simulink model "c00021M_harness"  (R2018a)
settings: Solver=ode3  StartTime=0.0  StopTime=10.0  RelTol=1e-3  EnableMultiTasking=on
undefined symbols (not defined in the file): b, DiscIntNeverNeededParam, J, K, L, PosMinimaW3, R, sigbuilder_block
(part 36 of 45)

== system c00021M_harness/M171/Physical/W/DC_Engine ==
  input : Inport
  (Inductance) : Gain  Gain=1/L
  (Inductance)1 : Gain  Gain=1/J
  Add : Sum  Inputs=-+-
  Add1 : Sum  Inputs=+-
  Damping : Gain  Gain=b
  Discrete-Time Integrator : DiscreteIntegrator  SampleTime=-1  ICPrevOutput=DiscIntNeverNeededParam  ICPrevScaledInput=DiscIntNeverNeededParam
  Discrete-Time Integrator1 : DiscreteIntegrator  SampleTime=-1  ICPrevOutput=DiscIntNeverNeededParam  ICPrevScaledInput=DiscIntNeverNeededParam
  Ke : Gain  Gain=K
  Kt : Gain  Gain=K
  Resistance : Gain  Gain=R
  Voltage : Gain  Gain=10
  Speed : Outport
  wires:
  (Inductance)/1 -> Discrete-Time Integrator/1
  Damping/1 -> Add1/2
  Discrete-Time Integrator1/1 -> Damping/1, Speed/1, Ke/1
  (Inductance)1/1 -> Discrete-Time Integrator1/1
  Add1/1 -> (Inductance)1/1
  Kt/1 -> Add1/1
  Ke/1 -> Add/3
  Resistance/1 -> Add/1
  Discrete-Time Integrator/1 -> Resistance/1, Kt/1
  Add/1 -> (Inductance)/1
  Voltage/1 -> Add/2
  input/1 -> Voltage/1

== system c00021M_harness/M171/Physical/W5/DC_Engine ==
  input : Inport
  (Inductance) : Gain  Gain=1/L
  (Inductance)1 : Gain  Gain=1/J
  Add : Sum  Inputs=-+-
  Add1 : Sum  Inputs=+-
  Damping : Gain  Gain=b
  Discrete-Time Integrator : DiscreteIntegrator  SampleTime=-1  ICPrevOutput=DiscIntNeverNeededParam  ICPrevScaledInput=DiscIntNeverNeededParam
  Discrete-Time Integrator1 : DiscreteIntegrator  SampleTime=-1  ICPrevOutput=DiscIntNeverNeededParam  ICPrevScaledInput=DiscIntNeverNeededParam
  Ke : Gain  Gain=K
  Kt : Gain  Gain=K
  Resistance : Gain  Gain=R
  Voltage : Gain  Gain=10
  Speed : Outport
  wires:
  input/1 -> Voltage/1
  Voltage/1 -> Add/2
  Add/1 -> (Inductance)/1
  (Inductance)/1 -> Discrete-Time Integrator/1
  Discrete-Time Integrator/1 -> Kt/1, Resistance/1
  Resistance/1 -> Add/1
  Ke/1 -> Add/3
  Kt/1 -> Add1/1
  Add1/1 -> (Inductance)1/1
  (Inductance)1/1 -> Discrete-Time Integrator1/1
  Discrete-Time Integrator1/1 -> Ke/1, Speed/1, Damping/1
  Damping/1 -> Add1/2

== system c00021M_harness/M171/Physical/W6/DC_Engine ==
  input : Inport
  (Inductance) : Gain  Gain=1/L
  (Inductance)1 : Gain  Gain=1/J
  Add : Sum  Inputs=-+-
  Add1 : Sum  Inputs=+-
  Damping : Gain  Gain=b
  Discrete-Time Integrator : DiscreteIntegrator  SampleTime=-1  ICPrevOutput=DiscIntNeverNeededParam  ICPrevScaledInput=DiscIntNeverNeededParam
  Discrete-Time Integrator1 : DiscreteIntegrator  SampleTime=-1  ICPrevOutput=DiscIntNeverNeededParam  ICPrevScaledInput=DiscIntNeverNeededParam
  Ke : Gain  Gain=K
  Kt : Gain  Gain=K
  Resistance : Gain  Gain=R
  Voltage : Gain  Gain=10
  Speed : Outport
  wires:
  Damping/1 -> Add1/2
  Discrete-Time Integrator1/1 -> Damping/1, Speed/1, Ke/1
  (Inductance)1/1 -> Discrete-Time Integrator1/1
  Add1/1 -> (Inductance)1/1
  Kt/1 -> Add1/1
  Ke/1 -> Add/3
  Resistance/1 -> Add/1
  Discrete-Time Integrator/1 -> Resistance/1, Kt/1
  (Inductance)/1 -> Discrete-Time Integrator/1
  Add/1 -> (Inductance)/1
  Voltage/1 -> Add/2
  input/1 -> Voltage/1

== system c00021M_harness/M172/Physical/W/DC_Engine ==
  input : Inport
  (Inductance) : Gain  Gain=1/L
  (Inductance)1 : Gain  Gain=1/J
  Add : Sum  Inputs=-+-
  Add1 : Sum  Inputs=+-
  Damping : Gain  Gain=b
  Discrete-Time Integrator : DiscreteIntegrator  SampleTime=-1  ICPrevOutput=DiscIntNeverNeededParam  ICPrevScaledInput=DiscIntNeverNeededParam
  Discrete-Time Integrator1 : DiscreteIntegrator  SampleTime=-1  ICPrevOutput=DiscIntNeverNeededParam  ICPrevScaledInput=DiscIntNeverNeededParam
  Ke : Gain  Gain=K
  Kt : Gain  Gain=K
  Resistance : Gain  Gain=R
  Voltage : Gain  Gain=10
  Speed : Outport
  wires:
  (Inductance)/1 -> Discrete-Time Integrator/1
  Damping/1 -> Add1/2
  Discrete-Time Integrator1/1 -> Damping/1, Speed/1, Ke/1
  (Inductance)1/1 -> Discrete-Time Integrator1/1
  Add1/1 -> (Inductance)1/1
  Kt/1 -> Add1/1
  Ke/1 -> Add/3
  Resistance/1 -> Add/1
  Discrete-Time Integrator/1 -> Resistance/1, Kt/1
  Add/1 -> (Inductance)/1
  Voltage/1 -> Add/2
  input/1 -> Voltage/1

== system c00021M_harness/M172/Physical/W5/DC_Engine ==
  input : Inport
  (Inductance) : Gain  Gain=1/L
  (Inductance)1 : Gain  Gain=1/J
  Add : Sum  Inputs=-+-
  Add1 : Sum  Inputs=+-
  Damping : Gain  Gain=b
  Discrete-Time Integrator : DiscreteIntegrator  SampleTime=-1  ICPrevOutput=DiscIntNeverNeededParam  ICPrevScaledInput=DiscIntNeverNeededParam
  Discrete-Time Integrator1 : DiscreteIntegrator  SampleTime=-1  ICPrevOutput=DiscIntNeverNeededParam  ICPrevScaledInput=DiscIntNeverNeededParam
  Ke : Gain  Gain=K
  Kt : Gain  Gain=K
  Resistance : Gain  Gain=R
  Voltage : Gain  Gain=10
  Speed : Outport
  wires:
  input/1 -> Voltage/1
  Voltage/1 -> Add/2
  Add/1 -> (Inductance)/1
  (Inductance)/1 -> Discrete-Time Integrator/1
  Discrete-Time Integrator/1 -> Kt/1, Resistance/1
  Resistance/1 -> Add/1
  Ke/1 -> Add/3
  Kt/1 -> Add1/1
  Add1/1 -> (Inductance)1/1
  (Inductance)1/1 -> Discrete-Time Integrator1/1
  Discrete-Time Integrator1/1 -> Ke/1, Speed/1, Damping/1
  Damping/1 -> Add1/2

== system c00021M_harness/M172/Physical/W6/DC_Engine ==
  input : Inport
  (Inductance) : Gain  Gain=1/L
  (Inductance)1 : Gain  Gain=1/J
  Add : Sum  Inputs=-+-
  Add1 : Sum  Inputs=+-
  Damping : Gain  Gain=b
  Discrete-Time Integrator : DiscreteIntegrator  SampleTime=-1  ICPrevOutput=DiscIntNeverNeededParam  ICPrevScaledInput=DiscIntNeverNeededParam
  Discrete-Time Integrator1 : DiscreteIntegrator  SampleTime=-1  ICPrevOutput=DiscIntNeverNeededParam  ICPrevScaledInput=DiscIntNeverNeededParam
  Ke : Gain  Gain=K
  Kt : Gain  Gain=K
  Resistance : Gain  Gain=R
  Voltage : Gain  Gain=10
  Speed : Outport
  wires:
  Damping/1 -> Add1/2
  Discrete-Time Integrator1/1 -> Damping/1, Speed/1, Ke/1
  (Inductance)1/1 -> Discrete-Time Integrator1/1
  Add1/1 -> (Inductance)1/1
  Kt/1 -> Add1/1
  Ke/1 -> Add/3
  Resistance/1 -> Add/1
  Discrete-Time Integrator/1 -> Resistance/1, Kt/1
  (Inductance)/1 -> Discrete-Time Integrator/1
  Add/1 -> (Inductance)/1
  Voltage/1 -> Add/2
  input/1 -> Voltage/1

== system c00021M_harness/M173/Physical/W/DC_Engine ==
  input : Inport
  (Inductance) : Gain  Gain=1/L
  (Inductance)1 : Gain  Gain=1/J
  Add : Sum  Inputs=-+-
  Add1 : Sum  Inputs=+-
  Damping : Gain  Gain=b
  Discrete-Time Integrator : DiscreteIntegrator  SampleTime=-1  ICPrevOutput=DiscIntNeverNeededParam  ICPrevScaledInput=DiscIntNeverNeededParam
  Discrete-Time Integrator1 : DiscreteIntegrator  SampleTime=-1  ICPrevOutput=DiscIntNeverNeededParam  ICPrevScaledInput=DiscIntNeverNeededParam
  Ke : Gain  Gain=K
  Kt : Gain  Gain=K
  Resistance : Gain  Gain=R
  Voltage : Gain  Gain=10
  Speed : Outport
  wires:
  (Inductance)/1 -> Discrete-Time Integrator/1
  Damping/1 -> Add1/2
  Discrete-Time Integrator1/1 -> Damping/1, Speed/1, Ke/1
  (Inductance)1/1 -> Discrete-Time Integrator1/1
  Add1/1 -> (Inductance)1/1
  Kt/1 -> Add1/1
  Ke/1 -> Add/3
  Resistance/1 -> Add/1
  Discrete-Time Integrator/1 -> Resistance/1, Kt/1
  Add/1 -> (Inductance)/1
  Voltage/1 -> Add/2
  input/1 -> Voltage/1

== system c00021M_harness/M173/Physical/W5/DC_Engine ==
  input : Inport
  (Inductance) : Gain  Gain=1/L
  (Inductance)1 : Gain  Gain=1/J
  Add : Sum  Inputs=-+-
  Add1 : Sum  Inputs=+-
  Damping : Gain  Gain=b
  Discrete-Time Integrator : DiscreteIntegrator  SampleTime=-1  ICPrevOutput=DiscIntNeverNeededParam  ICPrevScaledInput=DiscIntNeverNeededParam
  Discrete-Time Integrator1 : DiscreteIntegrator  SampleTime=-1  ICPrevOutput=DiscIntNeverNeededParam  ICPrevScaledInput=DiscIntNeverNeededParam
  Ke : Gain  Gain=K
  Kt : Gain  Gain=K
  Resistance : Gain  Gain=R
  Voltage : Gain  Gain=10
  Speed : Outport
  wires:
  input/1 -> Voltage/1
  Voltage/1 -> Add/2
  Add/1 -> (Inductance)/1
  (Inductance)/1 -> Discrete-Time Integrator/1
  Discrete-Time Integrator/1 -> Kt/1, Resistance/1
  Resistance/1 -> Add/1
  Ke/1 -> Add/3
  Kt/1 -> Add1/1
  Add1/1 -> (Inductance)1/1
  (Inductance)1/1 -> Discrete-Time Integrator1/1
  Discrete-Time Integrator1/1 -> Ke/1, Speed/1, Damping/1
  Damping/1 -> Add1/2

== system c00021M_harness/M173/Physical/W6/DC_Engine ==
  input : Inport
  (Inductance) : Gain  Gain=1/L
  (Inductance)1 : Gain  Gain=1/J
  Add : Sum  Inputs=-+-
  Add1 : Sum  Inputs=+-
  Damping : Gain  Gain=b
  Discrete-Time Integrator : DiscreteIntegrator  SampleTime=-1  ICPrevOutput=DiscIntNeverNeededParam  ICPrevScaledInput=DiscIntNeverNeededParam
  Discrete-Time Integrator1 : DiscreteIntegrator  SampleTime=-1  ICPrevOutput=DiscIntNeverNeededParam  ICPrevScaledInput=DiscIntNeverNeededParam
  Ke : Gain  Gain=K
  Kt : Gain  Gain=K
  Resistance : Gain  Gain=R
  Voltage : Gain  Gain=10
  Speed : Outport
  wires:
  Damping/1 -> Add1/2
  Discrete-Time Integrator1/1 -> Damping/1, Speed/1, Ke/1
  (Inductance)1/1 -> Discrete-Time Integrator1/1
  Add1/1 -> (Inductance)1/1
  Kt/1 -> Add1/1
  Ke/1 -> Add/3
  Resistance/1 -> Add/1
  Discrete-Time Integrator/1 -> Resistance/1, Kt/1
  (Inductance)/1 -> Discrete-Time Integrator/1
  Add/1 -> (Inductance)/1
  Voltage/1 -> Add/2
  input/1 -> Voltage/1

== stateflow chart c00021M_harness/CPSUT/Cyber/WL/Chart ==
  state Bajand_hasta_abajo
    entry: W = -1;
  state Bajando
    entry: W = -1;
  state Idle
    entry:W = 0;
  state Subiendo_hasta_arriba
    entry: W = 1;
  state Subiendo
    entry: W = 1;
  Subiendo -> Bajand_hasta_abajo [order 4] : [UI==4]
  Bajand_hasta_abajo -> Bajando [order 2] : [UI==3]
  Subiendo -> Bajando [order 3] : [UI==3]
  Bajando -> Bajand_hasta_abajo [order 2] : [UI==4]
  Idle -> Bajando [order 3] : [UI==3&&S>0]
  Subiendo_hasta_arriba -> Bajand_hasta_abajo [order 3] : [UI==4]
  Idle -> Bajand_hasta_abajo [order 4] : [UI==4&&S>0]
  Bajando -> Subiendo [order 3] : [UI==1]
  Subiendo_hasta_arriba -> Bajando [order 4] : [UI==3]
  Bajand_hasta_abajo -> Subiendo [order 4] : [UI==1]
  Bajand_hasta_abajo -> Idle [order 1] : [S<=0]
  Bajand_hasta_abajo -> Subiendo_hasta_arriba [order 3] : [UI==2]
  Bajando -> Idle [order 1] : [S<=0||UI==0]
  Bajando -> Subiendo_hasta_arriba [order 4] : [UI==2]
  (default) -> Idle
  Idle -> Subiendo_hasta_arriba [order 2] : [UI==2&&S<5]
  Idle -> Subiendo [order 1] : [UI == 1&&S<5]
  Subiendo -> Idle [order 1] : [S>=5||UI==0]
  Subiendo_hasta_arriba -> Idle [order 1] : [S >=5]
  Subiendo_hasta_arriba -> Subiendo [order 2] : [UI ==1]
  Subiendo -> Subiendo_hasta_arriba [order 2] : [UI==2]
  data: S input; UI input; W output double

== stateflow chart c00021M_harness/CPSUT/Cyber/WL2/Chart1 ==
  state Bajand_hasta_abajo
    entry: W = -1;
  state Bajando
    entry: W = -1;
  state Idle
    entry:W = 0;
  state Subiendo_hasta_arriba
    entry: W = 1;
  state Subiendo
    entry: W = 1;
  Subiendo -> Bajand_hasta_abajo [order 4] : [UI==4]
  Bajand_hasta_abajo -> Bajando [order 2] : [UI==3]
  Subiendo -> Bajando [order 3] : [UI==3]
  Bajando -> Bajand_hasta_abajo [order 2] : [UI==4]
  Idle -> Bajando [order 3] : [UI==3&&S>PosMinW3]
  Subiendo_hasta_arriba -> Bajand_hasta_abajo [order 3] : [UI==4]
  Idle -> Bajand_hasta_abajo [order 4] : [UI==4&&S>PosMinW3]
  Bajando -> Subiendo [order 3] : [UI==1]
  Subiendo_hasta_arriba -> Bajando [order 4] : [UI==3]
  Bajand_hasta_abajo -> Subiendo [order 4] : [UI==1]
  Bajand_hasta_abajo -> Idle [order 1] : [S<=PosMinW3]
  Bajand_hasta_abajo -> Subiendo_hasta_arriba [order 3] : [UI==2]
  Bajando -> Idle [order 1] : [S<=PosMinW3||UI==0]
  Bajando -> Subiendo_hasta_arriba [order 4] : [UI==2]
  (default) -> Idle
  Idle -> Subiendo_hasta_arriba [order 2] : [UI==2&&S<5]
  Idle -> Subiendo [order 1] : [UI == 1&&S<5]
  Subiendo -> Idle [order 1] : [S>=5||UI==0]
  Subiendo_hasta_arriba -> Idle [order 1] : [S >=5]
  Subiendo_hasta_arriba -> Subiendo [order 2] : [UI ==1]
  Subiendo -> Subiendo_hasta_arriba [order 2] : [UI==2]
  data: S input; UI input; W output double; PosMinW3 input

== stateflow chart c00021M_harness/CPSUT/Cyber/WL1/Chart1 ==
  state Bajand_hasta_abajo
    entry: W = -1;
  state Bajando
    entry: W = -1;
  state Idle
    entry:W = 0;
  state Subiendo_hasta_arriba
    entry: W = 1;
  state Subiendo
    entry: W = 1;
  Subiendo -> Bajand_hasta_abajo [order 4] : [UI==4]
  Bajand_hasta_abajo -> Bajando [order 2] : [UI==3]
  Subiendo -> Bajando [order 3] : [UI==3]
  Bajando -> Bajand_hasta_abajo [order 2] : [UI==4]
  Idle -> Bajando [order 3] : [UI==3&&S>0]
  Subiendo_hasta_arriba -> Bajand_hasta_abajo [order 3] : [UI==4]
  Idle -> Bajand_hasta_abajo [order 4] : [UI==4&&S>0]
  Bajando -> Subiendo [order 3] : [UI==1]
  Subiendo_hasta_arriba -> Bajando [order 4] : [UI==3]
  Bajand_hasta_abajo -> Subiendo [order 4] : [UI==1]
  Bajand_hasta_abajo -> Idle [order 1] : [S<=0]
  Bajand_hasta_abajo -> Subiendo_hasta_arriba [order 3] : [UI==2]
  Bajando -> Idle [order 1] : [S<=0||UI==0]
  Bajando -> Subiendo_hasta_arriba [order 4] : [UI==2]
  (default) -> Idle
  Idle -> Subiendo_hasta_arriba [order 2] : [UI==2&&S<5]
  Idle -> Subiendo [order 1] : [UI == 1&&S<5]
  Subiendo -> Idle [order 1] : [S>=5||UI==0]
  Subiendo_hasta_arriba -> Idle [order 1] : [S >=5]
  Subiendo_hasta_arriba -> Subiendo [order 2] : [UI ==1]
  Subiendo -> Subiendo_hasta_arriba [order 2] : [UI==2]
  data: S input; UI input; W output double

== stateflow chart c00021M_harness/M001/Cyber/WL/Chart ==
  state Bajand_hasta_abajo
    entry: W = -1;
  state Bajando
    entry: W = -1;
  state Idle
    entry:W = 0;
  state Subiendo_hasta_arriba
    entry: W = 1;
  state Subiendo
    entry: W = 1;
  Subiendo -> Bajand_hasta_abajo [order 4] : [UI==4]
  Bajand_hasta_abajo -> Bajando [order 2] : [UI==3]
  Subiendo -> Bajando [order 3] : [UI==3]
  Bajando -> Bajand_hasta_abajo [order 2] : [UI==4]
  Idle -> Bajando [order 3] : [UI==3&&S>0]
  Subiendo_hasta_arriba -> Bajand_hasta_abajo [order 3] : [UI==4]
  Idle -> Bajand_hasta_abajo [order 4] : [UI==4&&S>0]
  Bajando -> Subiendo [order 3] : [UI==1]
  Subiendo_hasta_arriba -> Bajando [order 4] : [UI==3]
  Bajand_hasta_abajo -> Subiendo [order 4] : [UI==1]
  Bajand_hasta_abajo -> Idle [order 1] : [S<=0]
  Bajand_hasta_abajo -> Subiendo_hasta_arriba [order 3] : [UI==2]
  Bajando -> Idle [order 1] : [S<=0||UI==0]
  Bajando -> Subiendo_hasta_arriba [order 4] : [UI==2]
  (default) -> Idle
  Idle -> Subiendo_hasta_arriba [order 2] : [UI==2&&S<5]
  Idle -> Subiendo [order 1] : [UI == 1&&S<5]
  Subiendo -> Idle [order 1] : [S>=5||UI==0]
  Subiendo_hasta_arriba -> Idle [order 1] : [S >=5]
  Subiendo_hasta_arriba -> Subiendo [order 2] : [UI ==1]
  Subiendo -> Subiendo_hasta_arriba [order 2] : [UI==2]
  data: S input; UI input; W output double

== stateflow chart c00021M_harness/M001/Cyber/WL1/Chart1 ==
  state Bajand_hasta_abajo
    entry: W = -1;
  state Bajando
    entry: W = -1;
  state Idle
    entry:W = 0;
  state Subiendo_hasta_arriba
    entry: W = 1;
  state Subiendo
    entry: W = 1;
  Subiendo -> Bajand_hasta_abajo [order 4] : [UI==4]
  Bajand_hasta_abajo -> Bajando [order 2] : [UI==3]
  Subiendo -> Bajando [order 3] : [UI==3]
  Bajando -> Bajand_hasta_abajo [order 2] : [UI==4]
  Idle -> Bajando [order 3] : [UI==3&&S>0]
  Subiendo_hasta_arriba -> Bajand_hasta_abajo [order 3] : [UI==4]
  Idle -> Bajand_hasta_abajo [order 4] : [UI==4&&S>0]
  Bajando -> Subiendo [order 3] : [UI==1]
  Subiendo_hasta_arriba -> Bajando [order 4] : [UI==3]
  Bajand_hasta_abajo -> Subiendo [order 4] : [UI==1]
  Bajand_hasta_abajo -> Idle [order 1] : [S<=0]
  Bajand_hasta_abajo -> Subiendo_hasta_arriba [order 3] : [UI==2]
  Bajando -> Idle [order 1] : [S<=0||UI==0]
  Bajando -> Subiendo_hasta_arriba [order 4] : [UI==2]
  (default) -> Idle
  Idle -> Subiendo_hasta_arriba [order 2] : [UI==2&&S<5]
  Idle -> Subiendo [order 1] : [UI == 1&&S<5]
  Subiendo -> Idle [order 1] : [S>=5||UI==0]
  Subiendo_hasta_arriba -> Idle [order 1] : [S >=5]
  Subiendo_hasta_arriba -> Subiendo [order 2] : [UI ==1]
  Subiendo -> Subiendo_hasta_arriba [order 2] : [UI==2]
  data: S input; UI input; W output double

== stateflow chart c00021M_harness/M001/Cyber/WL2/Chart1 ==
  state Bajand_hasta_abajo
    entry: W = -1;
  state Bajando
    entry: W = -1;
  state Idle
    entry:W = 0;
  state Subiendo_hasta_arriba
    entry: W = 1;
  state Subiendo
    entry: W = 1;
  Subiendo -> Bajand_hasta_abajo [order 4] : [UI==4]
  Bajand_hasta_abajo -> Bajando [order 2] : [UI==3]
  Subiendo -> Bajando [order 3] : [UI==3]
  Bajando -> Bajand_hasta_abajo [order 2] : [UI==4]
  Idle -> Bajando [order 3] : [UI==3&&S>PosMinW3]
  Subiendo_hasta_arriba -> Bajand_hasta_abajo [order 3] : [UI==4]
  Idle -> Bajand_hasta_abajo [order 4] : [UI==4&&S>PosMinW3]
  Bajando -> Subiendo [order 3] : [UI==1]
  Subiendo_hasta_arriba -> Bajando [order 4] : [UI==3]
  Bajand_hasta_abajo -> Subiendo [order 4] : [UI==1]
  Bajand_hasta_abajo -> Idle [order 1] : [S<=PosMinW3]
  Bajand_hasta_abajo -> Subiendo_hasta_arriba [order 3] : [UI==2]
  Bajando -> Idle [order 1] : [S<=PosMinW3||UI==0]
  Bajando -> Subiendo_hasta_arriba [order 4] : [UI==2]
  (default) -> Idle
  Idle -> Subiendo_hasta_arriba [order 2] : [UI==2&&S<5]
  Idle -> Subiendo [order 1] : [UI == 1&&S<5]
  Subiendo -> Idle [order 1] : [S>=5||UI==0]
  Subiendo_hasta_arriba -> Idle [order 1] : [S >=5]
  Subiendo_hasta_arriba -> Subiendo [order 2] : [UI ==1]
  Subiendo -> Subiendo_hasta_arriba [order 2] : [UI==2]
  data: S input; UI input; W output double; PosMinW3 input

== stateflow chart c00021M_harness/M002/Cyber/WL/Chart ==
  state Bajand_hasta_abajo
    entry: W = -1;
  state Bajando
    entry: W = -1;
  state Idle
    entry:W = 0;
  state Subiendo_hasta_arriba
    entry: W = 1;
  state Subiendo
    entry: W = 1;
  Subiendo -> Bajand_hasta_abajo [order 4] : [UI==4]
  Bajand_hasta_abajo -> Bajando [order 2] : [UI==3]
  Subiendo -> Bajando [order 3] : [UI==3]
  Bajando -> Bajand_hasta_abajo [order 2] : [UI==4]
  Idle -> Bajando [order 3] : [UI==3&&S>0]
  Subiendo_hasta_arriba -> Bajand_hasta_abajo [order 3] : [UI==4]
  Idle -> Bajand_hasta_abajo [order 4] : [UI==4&&S>0]
  Bajando -> Subiendo [order 3] : [UI==1]
  Subiendo_hasta_arriba -> Bajando [order 4] : [UI==3]
  Bajand_hasta_abajo -> Subiendo [order 4] : [UI==1]
  Bajand_hasta_abajo -> Idle [order 1] : [S<=0]
  Bajand_hasta_abajo -> Subiendo_hasta_arriba [order 3] : [UI==2]
  Bajando -> Idle [order 1] : [S<=0||UI==0]
  Bajando -> Subiendo_hasta_arriba [order 4] : [UI==2]
  (default) -> Idle
  Idle -> Subiendo_hasta_arriba [order 2] : [UI==2&&S<5]
  Idle -> Subiendo [order 1] : [UI == 1&&S<5]
  Subiendo -> Idle [order 1] : [S>=5||UI==0]
  Subiendo_hasta_arriba -> Idle [order 1] : [S >=5]
  Subiendo_hasta_arriba -> Subiendo [order 2] : [UI ==1]
  Subiendo -> Subiendo_hasta_arriba [order 2] : [UI==2]
  data: S input; UI input; W output double

== stateflow chart c00021M_harness/M002/Cyber/WL1/Chart1 ==
  state Bajand_hasta_abajo
    entry: W = -1;
  state Bajando
    entry: W = -1;
  state Idle
    entry:W = 0;
  state Subiendo_hasta_arriba
    entry: W = 1;
  state Subiendo
    entry: W = 1;
  Subiendo -> Bajand_hasta_abajo [order 4] : [UI==4]
  Bajand_hasta_abajo -> Bajando [order 2] : [UI==3]
  Subiendo -> Bajando [order 3] : [UI==3]
  Bajando -> Bajand_hasta_abajo [order 2] : [UI==4]
  Idle -> Bajando [order 3] : [UI==3&&S>0]
  Subiendo_hasta_arriba -> Bajand_hasta_abajo [order 3] : [UI==4]
  Idle -> Bajand_hasta_abajo [order 4] : [UI==4&&S>0]
  Bajando -> Subiendo [order 3] : [UI==1]
  Subiendo_hasta_arriba -> Bajando [order 4] : [UI==3]
  Bajand_hasta_abajo -> Subiendo [order 4] : [UI==1]
  Bajand_hasta_abajo -> Idle [order 1] : [S<=0]
  Bajand_hasta_abajo -> Subiendo_hasta_arriba [order 3] : [UI==2]
  Bajando -> Idle [order 1] : [S<=0||UI==0]
  Bajando -> Subiendo_hasta_arriba [order 4] : [UI==2]
  (default) -> Idle
  Idle -> Subiendo_hasta_arriba [order 2] : [UI==2&&S<5]
  Idle -> Subiendo [order 1] : [UI == 1&&S<5]
  Subiendo -> Idle [order 1] : [S>=5||UI==0]
  Subiendo_hasta_arriba -> Idle [order 1] : [S >=5]
  Subiendo_hasta_arriba -> Subiendo [order 2] : [UI ==1]
  Subiendo -> Subiendo_hasta_arriba [order 2] : [UI==2]
  data: S input; UI input; W output double

== stateflow chart c00021M_harness/M002/Cyber/WL2/Chart1 ==
  state Bajand_hasta_abajo
    entry: W = -1;
  state Bajando
    entry: W = -1;
  state Idle
    entry:W = 0;
  state Subiendo_hasta_arriba
    entry: W = 1;
  state Subiendo
    entry: W = 1;
  Subiendo -> Bajand_hasta_abajo [order 4] : [UI==4]
  Bajand_hasta_abajo -> Bajando [order 2] : [UI==3]
  Subiendo -> Bajando [order 3] : [UI==3]
  Bajando -> Bajand_hasta_abajo [order 2] : [UI==4]
  Idle -> Bajando [order 3] : [UI==3&&S>PosMinW3]
  Subiendo_hasta_arriba -> Bajand_hasta_abajo [order 3] : [UI==4]
  Idle -> Bajand_hasta_abajo [order 4] : [UI==4&&S>PosMinW3]
  Bajando -> Subiendo [order 3] : [UI==1]
  Subiendo_hasta_arriba -> Bajando [order 4] : [UI==3]
  Bajand_hasta_abajo -> Subiendo [order 4] : [UI==1]
  Bajand_hasta_abajo -> Idle [order 1] : [S<=PosMinW3]
  Bajand_hasta_abajo -> Subiendo_hasta_arriba [order 3] : [UI==2]
  Bajando -> Idle [order 1] : [S<=PosMinW3||UI==0]
  Bajando -> Subiendo_hasta_arriba [order 4] : [UI==2]
  (default) -> Idle
  Idle -> Subiendo_hasta_arriba [order 2] : [UI==2&&S<5]
  Idle -> Subiendo [order 1] : [UI == 1&&S<5]
  Subiendo -> Idle [order 1] : [S>=5||UI==0]
  Subiendo_hasta_arriba -> Idle [order 1] : [S >=5]
  Subiendo_hasta_arriba -> Subiendo [order 2] : [UI ==1]
  Subiendo -> Subiendo_hasta_arriba [order 2] : [UI==2]
  data: S input; UI input; W output double; PosMinW3 input

== stateflow chart c00021M_harness/M003/Cyber/WL/Chart ==
  state Bajand_hasta_abajo
    entry: W = -1;
  state Bajando
    entry: W = -1;
  state Idle
    entry:W = 0;
  state Subiendo_hasta_arriba
    entry: W = 1;
  state Subiendo
    entry: W = 1;
  Subiendo -> Bajand_hasta_abajo [order 4] : [UI==4]
  Bajand_hasta_abajo -> Bajando [order 2] : [UI==3]
  Subiendo -> Bajando [order 3] : [UI==3]
  Bajando -> Bajand_hasta_abajo [order 2] : [UI==4]
  Idle -> Bajando [order 3] : [UI==3&&S>0]
  Subiendo_hasta_arriba -> Bajand_hasta_abajo [order 3] : [UI==4]
  Idle -> Bajand_hasta_abajo [order 4] : [UI==4&&S>0]
  Bajando -> Subiendo [order 3] : [UI==1]
  Subiendo_hasta_arriba -> Bajando [order 4] : [UI==3]
  Bajand_hasta_abajo -> Subiendo [order 4] : [UI==1]
  Bajand_hasta_abajo -> Idle [order 1] : [S<=0]
  Bajand_hasta_abajo -> Subiendo_hasta_arriba [order 3] : [UI==2]
  Bajando -> Idle [order 1] : [S<=0||UI==0]
  Bajando -> Subiendo_hasta_arriba [order 4] : [UI==2]
  (default) -> Idle
  Idle -> Subiendo_hasta_arriba [order 2] : [UI==2&&S<5]
  Idle -> Subiendo [order 1] : [UI == 1&&S<5]
  Subiendo -> Idle [order 1] : [S>=5||UI==0]
  Subiendo_hasta_arriba -> Idle [order 1] : [S >=5]
  Subiendo_hasta_arriba -> Subiendo [order 2] : [UI ==1]
  Subiendo -> Subiendo_hasta_arriba [order 2] : [UI==2]
  data: S input; UI input; W output double

== stateflow chart c00021M_harness/M003/Cyber/WL1/Chart1 ==
  state Bajand_hasta_abajo
    entry: W = -1;
  state Bajando
    entry: W = -1;
  state Idle
    entry:W = 0;
  state Subiendo_hasta_arriba
    entry: W = 1;
  state Subiendo
    entry: W = 1;
  Subiendo -> Bajand_hasta_abajo [order 4] : [UI==4]
  Bajand_hasta_abajo -> Bajando [order 2] : [UI==3]
  Subiendo -> Bajando [order 3] : [UI==3]
  Bajando -> Bajand_hasta_abajo [order 2] : [UI==4]
  Idle -> Bajando [order 3] : [UI==3&&S>0]
  Subiendo_hasta_arriba -> Bajand_hasta_abajo [order 3] : [UI==4]
  Idle -> Bajand_hasta_abajo [order 4] : [UI==4&&S>0]
  Bajando -> Subiendo [order 3] : [UI==1]
  Subiendo_hasta_arriba -> Bajando [order 4] : [UI==3]
  Bajand_hasta_abajo -> Subiendo [order 4] : [UI==1]
  Bajand_hasta_abajo -> Idle [order 1] : [S<=0]
  Bajand_hasta_abajo -> Subiendo_hasta_arriba [order 3] : [UI==2]
  Bajando -> Idle [order 1] : [S<=0||UI==0]
  Bajando -> Subiendo_hasta_arriba [order 4] : [UI==2]
  (default) -> Idle
  Idle -> Subiendo_hasta_arriba [order 2] : [UI==2&&S<5]
  Idle -> Subiendo [order 1] : [UI == 1&&S<5]
  Subiendo -> Idle [order 1] : [S>=5||UI==0]
  Subiendo_hasta_arriba -> Idle [order 1] : [S >=5]
  Subiendo_hasta_arriba -> Subiendo [order 2] : [UI ==1]
  Subiendo -> Subiendo_hasta_arriba [order 2] : [UI==2]
  data: S input; UI input; W output double

== stateflow chart c00021M_harness/M003/Cyber/WL2/Chart1 ==
  state Bajand_hasta_abajo
    entry: W = -1;
  state Bajando
    entry: W = -1;
  state Idle
    entry:W = 0;
  state Subiendo_hasta_arriba
    entry: W = 1;
  state Subiendo
    entry: W = 1;
  Subiendo -> Bajand_hasta_abajo [order 4] : [UI==4]
  Bajand_hasta_abajo -> Bajando [order 2] : [UI==3]
  Subiendo -> Bajando [order 3] : [UI==3]
  Bajando -> Bajand_hasta_abajo [order 2] : [UI==4]
  Idle -> Bajando [order 3] : [UI==3&&S>PosMinW3]
  Subiendo_hasta_arriba -> Bajand_hasta_abajo [order 3] : [UI==4]
  Idle -> Bajand_hasta_abajo [order 4] : [UI==4&&S>PosMinW3]
  Bajando -> Subiendo [order 3] : [UI==1]
  Subiendo_hasta_arriba -> Bajando [order 4] : [UI==3]
  Bajand_hasta_abajo -> Subiendo [order 4] : [UI==1]
  Bajand_hasta_abajo -> Idle [order 1] : [S<=PosMinW3]
  Bajand_hasta_abajo -> Subiendo_hasta_arriba [order 3] : [UI==2]
  Bajando -> Idle [order 1] : [S<=PosMinW3||UI==0]
  Bajando -> Subiendo_hasta_arriba [order 4] : [UI==2]
  (default) -> Idle
  Idle -> Subiendo_hasta_arriba [order 2] : [UI==2&&S<5]
  Idle -> Subiendo [order 1] : [UI == 1&&S<5]
  Subiendo -> Idle [order 1] : [S>=5||UI==0]
  Subiendo_hasta_arriba -> Idle [order 1] : [S >=5]
  Subiendo_hasta_arriba -> Subiendo [order 2] : [UI ==1]
  Subiendo -> Subiendo_hasta_arriba [order 2] : [UI==2]
  data: S input; UI input; W output double; PosMinW3 input

== stateflow chart c00021M_harness/M004/Cyber/WL/Chart ==
  state Bajand_hasta_abajo
    entry: W = -1;
  state Bajando
    entry: W = -1;
  state Idle
    entry:W = 0;
  state Subiendo_hasta_arriba
    entry: W = 1;
  state Subiendo
    entry: W = 1;
  Subiendo -> Bajand_hasta_abajo [order 4] : [UI==4]
  Bajand_hasta_abajo -> Bajando [order 2] : [UI==3]
  Subiendo -> Bajando [order 3] : [UI==3]
  Bajando -> Bajand_hasta_abajo [order 2] : [UI==4]
  Idle -> Bajando [order 3] : [UI==3&&S>0]
  Subiendo_hasta_arriba -> Bajand_hasta_abajo [order 3] : [UI==4]
  Idle -> Bajand_hasta_abajo [order 4] : [UI==4&&S>0]
  Bajando -> Subiendo [order 3] : [UI==1]
  Subiendo_hasta_arriba -> Bajando [order 4] : [UI==3]
  Bajand_hasta_abajo -> Subiendo [order 4] : [UI==1]
  Bajand_hasta_abajo -> Idle [order 1] : [S<=0]
  Bajand_hasta_abajo -> Subiendo_hasta_arriba [order 3] : [UI==2]
  Bajando -> Idle [order 1] : [S<=0||UI==0]
  Bajando -> Subiendo_hasta_arriba [order 4] : [UI==2]
  (default) -> Idle
  Idle -> Subiendo_hasta_arriba [order 2] : [UI==2&&S<5]
  Idle -> Subiendo [order 1] : [UI == 1&&S<5]
  Subiendo -> Idle [order 1] : [S>=5||UI==0]
  Subiendo_hasta_arriba -> Idle [order 1] : [S >=5]
  Subiendo_hasta_arriba -> Subiendo [order 2] : [UI ==1]
  Subiendo -> Subiendo_hasta_arriba [order 2] : [UI==2]
  data: S input; UI input; W output double

== stateflow chart c00021M_harness/M004/Cyber/WL1/Chart1 ==
  state Bajand_hasta_abajo
    entry: W = -1;
  state Bajando
    entry: W = -1;
  state Idle
    entry:W = 0;
  state Subiendo_hasta_arriba
    entry: W = 1;
  state Subiendo
    entry: W = 1;
  Subiendo -> Bajand_hasta_abajo [order 4] : [UI==4]
  Bajand_hasta_abajo -> Bajando [order 2] : [UI==3]
  Subiendo -> Bajando [order 3] : [UI==3]
  Bajando -> Bajand_hasta_abajo [order 2] : [UI==4]
  Idle -> Bajando [order 3] : [UI==3&&S>0]
  Subiendo_hasta_arriba -> Bajand_hasta_abajo [order 3] : [UI==4]
  Idle -> Bajand_hasta_abajo [order 4] : [UI==4&&S>0]
  Bajando -> Subiendo [order 3] : [UI==1]
  Subiendo_hasta_arriba -> Bajando [order 4] : [UI==3]
  Bajand_hasta_abajo -> Subiendo [order 4] : [UI==1]
  Bajand_hasta_abajo -> Idle [order 1] : [S<=0]
  Bajand_hasta_abajo -> Subiendo_hasta_arriba [order 3] : [UI==2]
  Bajando -> Idle [order 1] : [S<=0||UI==0]
  Bajando -> Subiendo_hasta_arriba [order 4] : [UI==2]
  (default) -> Idle
  Idle -> Subiendo_hasta_arriba [order 2] : [UI==2&&S<5]
  Idle -> Subiendo [order 1] : [UI == 1&&S<5]
  Subiendo -> Idle [order 1] : [S>=5||UI==0]
  Subiendo_hasta_arriba -> Idle [order 1] : [S >=5]
  Subiendo_hasta_arriba -> Subiendo [order 2] : [UI ==1]
  Subiendo -> Subiendo_hasta_arriba [order 2] : [UI==2]
  data: S input; UI input; W output double

== stateflow chart c00021M_harness/M004/Cyber/WL2/Chart1 ==
  state Bajand_hasta_abajo
    entry: W = -1;
  state Bajando
    entry: W = -1;
  state Idle
    entry:W = 0;
  state Subiendo_hasta_arriba
    entry: W = 1;
  state Subiendo
    entry: W = 1;
  Subiendo -> Bajand_hasta_abajo [order 4] : [UI==4]
  Bajand_hasta_abajo -> Bajando [order 2] : [UI==3]
  Subiendo -> Bajando [order 3] : [UI==3]
  Bajando -> Bajand_hasta_abajo [order 2] : [UI==4]
  Idle -> Bajando [order 3] : [UI==3&&S>PosMinW3]
  Subiendo_hasta_arriba -> Bajand_hasta_abajo [order 3] : [UI==4]
  Idle -> Bajand_hasta_abajo [order 4] : [UI==4&&S>PosMinW3]
  Bajando -> Subiendo [order 3] : [UI==1]
  Subiendo_hasta_arriba -> Bajando [order 4] : [UI==3]
  Bajand_hasta_abajo -> Subiendo [order 4] : [UI==1]
  Bajand_hasta_abajo -> Idle [order 1] : [S<=PosMinW3]
  Bajand_hasta_abajo -> Subiendo_hasta_arriba [order 3] : [UI==2]
  Bajando -> Idle [order 1] : [S<=PosMinW3||UI==0]
  Bajando -> Subiendo_hasta_arriba [order 4] : [UI==2]
  (default) -> Idle
  Idle -> Subiendo_hasta_arriba [order 2] : [UI==2&&S<5]
  Idle -> Subiendo [order 1] : [UI == 1&&S<5]
  Subiendo -> Idle [order 1] : [S>=5||UI==0]
  Subiendo_hasta_arriba -> Idle [order 1] : [S >=5]
  Subiendo_hasta_arriba -> Subiendo [order 2] : [UI ==1]
  Subiendo -> Subiendo_hasta_arriba [order 2] : [UI==2]
  data: S input; UI input; W output double; PosMinW3 input

== stateflow chart c00021M_harness/M005/Cyber/WL/Chart ==
  state Bajand_hasta_abajo
    entry: W = -1;
  state Bajando
    entry: W = -1;
  state Idle
    entry:W = 0;
  state Subiendo_hasta_arriba
    entry: W = 1;
  state Subiendo
    entry: W = 1;
  Subiendo -> Bajand_hasta_abajo [order 4] : [UI==4]
  Bajand_hasta_abajo -> Bajando [order 2] : [UI==3]
  Subiendo -> Bajando [order 3] : [UI==3]
  Bajando -> Bajand_hasta_abajo [order 2] : [UI==4]
  Idle -> Bajando [order 3] : [UI==3&&S>0]
  Subiendo_hasta_arriba -> Bajand_hasta_abajo [order 3] : [UI==4]
  Idle -> Bajand_hasta_abajo [order 4] : [UI==4&&S>0]
  Bajando -> Subiendo [order 3] : [UI==1]
  Subiendo_hasta_arriba -> Bajando [order 4] : [UI==3]
  Bajand_hasta_abajo -> Subiendo [order 4] : [UI==1]
  Bajand_hasta_abajo -> Idle [order 1] : [S<=0]
  Bajand_hasta_abajo -> Subiendo_hasta_arriba [order 3] : [UI==2]
  Bajando -> Idle [order 1] : [S<=0||UI==0]
  Bajando -> Subiendo_hasta_arriba [order 4] : [UI==2]
  (default) -> Idle
  Idle -> Subiendo_hasta_arriba [order 2] : [UI==2&&S<5]
  Idle -> Subiendo [order 1] : [UI == 1&&S<5]
  Subiendo -> Idle [order 1] : [S>=5||UI==0]
  Subiendo_hasta_arriba -> Idle [order 1] : [S >=5]
  Subiendo_hasta_arriba -> Subiendo [order 2] : [UI ==1]
  Subiendo -> Subiendo_hasta_arriba [order 2] : [UI==2]
  data: S input; UI input; W output double

== stateflow chart c00021M_harness/M005/Cyber/WL1/Chart1 ==
  state Bajand_hasta_abajo
    entry: W = -1;
  state Bajando
    entry: W = -1;
  state Idle
    entry:W = 0;
  state Subiendo_hasta_arriba
    entry: W = 1;
  state Subiendo
    entry: W = 1;
  Subiendo -> Bajand_hasta_abajo [order 4] : [UI==4]
  Bajand_hasta_abajo -> Bajando [order 2] : [UI==3]
  Subiendo -> Bajando [order 3] : [UI==3]
  Bajando -> Bajand_hasta_abajo [order 2] : [UI==4]
  Idle -> Bajando [order 3] : [UI==3&&S>0]
  Subiendo_hasta_arriba -> Bajand_hasta_abajo [order 3] : [UI==4]
  Idle -> Bajand_hasta_abajo [order 4] : [UI==4&&S>0]
  Bajando -> Subiendo [order 3] : [UI==1]
  Subiendo_hasta_arriba -> Bajando [order 4] : [UI==3]
  Bajand_hasta_abajo -> Subiendo [order 4] : [UI==1]
  Bajand_hasta_abajo -> Idle [order 1] : [S<=0]
  Bajand_hasta_abajo -> Subiendo_hasta_arriba [order 3] : [UI==2]
  Bajando -> Idle [order 1] : [S<=0||UI==0]
  Bajando -> Subiendo_hasta_arriba [order 4] : [UI==2]
  (default) -> Idle
  Idle -> Subiendo_hasta_arriba [order 2] : [UI==2&&S<5]
  Idle -> Subiendo [order 1] : [UI == 1&&S<5]
  Subiendo -> Idle [order 1] : [S>=5||UI==0]
  Subiendo_hasta_arriba -> Idle [order 1] : [S >=5]
  Subiendo_hasta_arriba -> Subiendo [order 2] : [UI ==1]
  Subiendo -> Subiendo_hasta_arriba [order 2] : [UI==2]
  data: S input; UI input; W output double

== stateflow chart c00021M_harness/M005/Cyber/WL2/Chart1 ==
  state Bajand_hasta_abajo
    entry: W = -1;
  state Bajando
    entry: W = -1;
  state Idle
    entry:W = 0;
  state Subiendo_hasta_arriba
    entry: W = 1;
  state Subiendo
    entry: W = 1;
  Subiendo -> Bajand_hasta_abajo [order 4] : [UI==4]
  Bajand_hasta_abajo -> Bajando [order 2] : [UI==3]
  Subiendo -> Bajando [order 3] : [UI==3]
  Bajando -> Bajand_hasta_abajo [order 2] : [UI==4]
  Idle -> Bajando [order 3] : [UI==3&&S>PosMinW3]
  Subiendo_hasta_arriba -> Bajand_hasta_abajo [order 3] : [UI==4]
  Idle -> Bajand_hasta_abajo [order 4] : [UI==4&&S>PosMinW3]
  Bajando -> Subiendo [order 3] : [UI==1]
  Subiendo_hasta_arriba -> Bajando [order 4] : [UI==3]
  Bajand_hasta_abajo -> Subiendo [order 4] : [UI==1]
  Bajand_hasta_abajo -> Idle [order 1] : [S<=PosMinW3]
  Bajand_hasta_abajo -> Subiendo_hasta_arriba [order 3] : [UI==2]
  Bajando -> Idle [order 1] : [S<=PosMinW3||UI==0]
  Bajando -> Subiendo_hasta_arriba [order 4] : [UI==2]
  (default) -> Idle
  Idle -> Subiendo_hasta_arriba [order 2] : [UI==2&&S<5]
  Idle -> Subiendo [order 1] : [UI == 1&&S<5]
  Subiendo -> Idle [order 1] : [S>=5||UI==0]
  Subiendo_hasta_arriba -> Idle [order 1] : [S >=5]
  Subiendo_hasta_arriba -> Subiendo [order 2] : [UI ==1]
  Subiendo -> Subiendo_hasta_arriba [order 2] : [UI==2]
  data: S input; UI input; W output double; PosMinW3 input

== stateflow chart c00021M_harness/M006/Cyber/WL/Chart ==
  state Bajand_hasta_abajo
    entry: W = -1;
  state Bajando
    entry: W = -1;
  state Idle
    entry:W = 0;
  state Subiendo_hasta_arriba
    entry: W = 1;
  state Subiendo
    entry: W = 1;
  Subiendo -> Bajand_hasta_abajo [order 4] : [UI==4]
  Bajand_hasta_abajo -> Bajando [order 2] : [UI==3]
  Subiendo -> Bajando [order 3] : [UI==3]
  Bajando -> Bajand_hasta_abajo [order 2] : [UI==4]
  Idle -> Bajando [order 3] : [UI==3&&S>0]
  Subiendo_hasta_arriba -> Bajand_hasta_abajo [order 3] : [UI==4]
  Idle -> Bajand_hasta_abajo [order 4] : [UI==4&&S>0]
  Bajando -> Subiendo [order 3] : [UI==1]
  Subiendo_hasta_arriba -> Bajando [order 4] : [UI==3]
  Bajand_hasta_abajo -> Subiendo [order 4] : [UI==1]
  Bajand_hasta_abajo -> Idle [order 1] : [S<=0]
  Bajand_hasta_abajo -> Subiendo_hasta_arriba [order 3] : [UI==2]
  Bajando -> Idle [order 1] : [S<=0||UI==0]
  Bajando -> Subiendo_hasta_arriba [order 4] : [UI==2]
  (default) -> Idle
  Idle -> Subiendo_hasta_arriba [order 2] : [UI==2&&S<5]
  Idle -> Subiendo [order 1] : [UI == 1&&S<5]
  Subiendo -> Idle [order 1] : [S>=5||UI==0]
  Subiendo_hasta_arriba -> Idle [order 1] : [S >=5]
  Subiendo_hasta_arriba -> Subiendo [order 2] : [UI ==1]
  Subiendo -> Subiendo_hasta_arriba [order 2] : [UI==2]
  data: S input; UI input; W output double

== stateflow chart c00021M_harness/M006/Cyber/WL1/Chart1 ==
  state Bajand_hasta_abajo
    entry: W = -1;
  state Bajando
    entry: W = -1;
  state Idle
    entry:W = 0;
  state Subiendo_hasta_arriba
    entry: W = 1;
  state Subiendo
    entry: W = 1;
  Subiendo -> Bajand_hasta_abajo [order 4] : [UI==4]
  Bajand_hasta_abajo -> Bajando [order 2] : [UI==3]
  Subiendo -> Bajando [order 3] : [UI==3]
  Bajando -> Bajand_hasta_abajo [order 2] : [UI==4]
  Idle -> Bajando [order 3] : [UI==3&&S>0]
  Subiendo_hasta_arriba -> Bajand_hasta_abajo [order 3] : [UI==4]
  Idle -> Bajand_hasta_abajo [order 4] : [UI==4&&S>0]
  Bajando -> Subiendo [order 3] : [UI==1]
  Subiendo_hasta_arriba -> Bajando [order 4] : [UI==3]
  Bajand_hasta_abajo -> Subiendo [order 4] : [UI==1]
  Bajand_hasta_abajo -> Idle [order 1] : [S<=0]
  Bajand_hasta_abajo -> Subiendo_hasta_arriba [order 3] : [UI==2]
  Bajando -> Idle [order 1] : [S<=0||UI==0]
  Bajando -> Subiendo_hasta_arriba [order 4] : [UI==2]
  (default) -> Idle
  Idle -> Subiendo_hasta_arriba [order 2] : [UI==2&&S<5]
  Idle -> Subiendo [order 1] : [UI == 1&&S<5]
  Subiendo -> Idle [order 1] : [S>=5||UI==0]
  Subiendo_hasta_arriba -> Idle [order 1] : [S >=5]
  Subiendo_hasta_arriba -> Subiendo [order 2] : [UI ==1]
  Subiendo -> Subiendo_hasta_arriba [order 2] : [UI==2]
  data: S input; UI input; W output double

== stateflow chart c00021M_harness/M006/Cyber/WL2/Chart1 ==
  state Bajand_hasta_abajo
    entry: W = -1;
  state Bajando
    entry: W = -1;
  state Idle
    entry:W = 0;
  state Subiendo_hasta_arriba
    entry: W = 1;
  state Subiendo
    entry: W = 1;
  Subiendo -> Bajand_hasta_abajo [order 4] : [UI==4]
  Bajand_hasta_abajo -> Bajando [order 2] : [UI==3]
  Subiendo -> Bajando [order 3] : [UI==3]
  Bajando -> Bajand_hasta_abajo [order 2] : [UI==4]
  Idle -> Bajando [order 3] : [UI==3&&S>PosMinW3]
  Subiendo_hasta_arriba -> Bajand_hasta_abajo [order 3] : [UI==4]
  Idle -> Bajand_hasta_abajo [order 4] : [UI==4&&S>PosMinW3]
  Bajando -> Subiendo [order 3] : [UI==1]
  Subiendo_hasta_arriba -> Bajando [order 4] : [UI==3]
  Bajand_hasta_abajo -> Subiendo [order 4] : [UI==1]
  Bajand_hasta_abajo -> Idle [order 1] : [S<=PosMinW3]
  Bajand_hasta_abajo -> Subiendo_hasta_arriba [order 3] : [UI==2]
  Bajando -> Idle [order 1] : [S<=PosMinW3||UI==0]
  Bajando -> Subiendo_hasta_arriba [order 4] : [UI==2]
  (default) -> Idle
  Idle -> Subiendo_hasta_arriba [order 2] : [UI==2&&S<5]
  Idle -> Subiendo [order 1] : [UI == 1&&S<5]
  Subiendo -> Idle [order 1] : [S>=5||UI==0]
  Subiendo_hasta_arriba -> Idle [order 1] : [S >=5]
  Subiendo_hasta_arriba -> Subiendo [order 2] : [UI ==1]
  Subiendo -> Subiendo_hasta_arriba [order 2] : [UI==2]
  data: S input; UI input; W output double; PosMinW3 input

== stateflow chart c00021M_harness/M007/Cyber/WL/Chart ==
  state Bajand_hasta_abajo
    entry: W = -1;
  state Bajando
    entry: W = -1;
  state Idle
    entry:W = 0;
  state Subiendo_hasta_arriba
    entry: W = 1;
  state Subiendo
    entry: W = 1;
  Subiendo -> Bajand_hasta_abajo [order 4] : [UI==4]
  Bajand_hasta_abajo -> Bajando [order 2] : [UI==3]
  Subiendo -> Bajando [order 3] : [UI==3]
  Bajando -> Bajand_hasta_abajo [order 2] : [UI==4]
  Idle -> Bajando [order 3] : [UI==3&&S>0]
  Subiendo_hasta_arriba -> Bajand_hasta_abajo [order 3] : [UI==4]
  Idle -> Bajand_hasta_abajo [order 4] : [UI==4&&S>0]
  Bajando -> Subiendo [order 3] : [UI==1]
  Subiendo_hasta_arriba -> Bajando [order 4] : [UI==3]
  Bajand_hasta_abajo -> Subiendo [order 4] : [UI==1]
  Bajand_hasta_abajo -> Idle [order 1] : [S<=0]
  Bajand_hasta_abajo -> Subiendo_hasta_arriba [order 3] : [UI==2]
  Bajando -> Idle [order 1] : [S<=0||UI==0]
  Bajando -> Subiendo_hasta_arriba [order 4] : [UI==2]
  (default) -> Idle
  Idle -> Subiendo_hasta_arriba [order 2] : [UI==2&&S<5]
  Idle -> Subiendo [order 1] : [UI == 1&&S<5]
  Subiendo -> Idle [order 1] : [S>=5||UI==0]
  Subiendo_hasta_arriba -> Idle [order 1] : [S >=5]
  Subiendo_hasta_arriba -> Subiendo [order 2] : [UI ==1]
  Subiendo -> Subiendo_hasta_arriba [order 2] : [UI==2]
  data: S input; UI input; W output double

== stateflow chart c00021M_harness/M007/Cyber/WL1/Chart1 ==
  state Bajand_hasta_abajo
    entry: W = -1;
  state Bajando
    entry: W = -1;
  state Idle
    entry:W = 0;
  state Subiendo_hasta_arriba
    entry: W = 1;
  state Subiendo
    entry: W = 1;
  Subiendo -> Bajand_hasta_abajo [order 4] : [UI==4]
  Bajand_hasta_abajo -> Bajando [order 2] : [UI==3]
  Subiendo -> Bajando [order 3] : [UI==3]
  Bajando -> Bajand_hasta_abajo [order 2] : [UI==4]
  Idle -> Bajando [order 3] : [UI==3&&S>0]
  Subiendo_hasta_arriba -> Bajand_hasta_abajo [order 3] : [UI==4]
  Idle -> Bajand_hasta_abajo [order 4] : [UI==4&&S>0]
  Bajando -> Subiendo [order 3] : [UI==1]
  Subiendo_hasta_arriba -> Bajando [order 4] : [UI==3]
  Bajand_hasta_abajo -> Subiendo [order 4] : [UI==1]
  Bajand_hasta_abajo -> Idle [order 1] : [S<=0]
  Bajand_hasta_abajo -> Subiendo_hasta_arriba [order 3] : [UI==2]
  Bajando -> Idle [order 1] : [S<=0||UI==0]
  Bajando -> Subiendo_hasta_arriba [order 4] : [UI==2]
  (default) -> Idle
  Idle -> Subiendo_hasta_arriba [order 2] : [UI==2&&S<5]
  Idle -> Subiendo [order 1] : [UI == 1&&S<5]
  Subiendo -> Idle [order 1] : [S>=5||UI==0]
  Subiendo_hasta_arriba -> Idle [order 1] : [S >=5]
  Subiendo_hasta_arriba -> Subiendo [order 2] : [UI ==1]
  Subiendo -> Subiendo_hasta_arriba [order 2] : [UI==2]
  data: S input; UI input; W output double

== stateflow chart c00021M_harness/M007/Cyber/WL2/Chart1 ==
  state Bajand_hasta_abajo
    entry: W = -1;
  state Bajando
    entry: W = -1;
  state Idle
    entry:W = 0;
  state Subiendo_hasta_arriba
    entry: W = 1;
  state Subiendo
    entry: W = 1;
  Subiendo -> Bajand_hasta_abajo [order 4] : [UI==4]
  Bajand_hasta_abajo -> Bajando [order 2] : [UI==3]
  Subiendo -> Bajando [order 3] : [UI==3]
  Bajando -> Bajand_hasta_abajo [order 2] : [UI==4]
  Idle -> Bajando [order 3] : [UI==3&&S>PosMinW3]
  Subiendo_hasta_arriba -> Bajand_hasta_abajo [order 3] : [UI==4]
  Idle -> Bajand_hasta_abajo [order 4] : [UI==4&&S>PosMinW3]
  Bajando -> Subiendo [order 3] : [UI==1]
  Subiendo_hasta_arriba -> Bajando [order 4] : [UI==3]
  Bajand_hasta_abajo -> Subiendo [order 4] : [UI==1]
  Bajand_hasta_abajo -> Idle [order 1] : [S<=PosMinW3]
  Bajand_hasta_abajo -> Subiendo_hasta_arriba [order 3] : [UI==2]
  Bajando -> Idle [order 1] : [S<=PosMinW3||UI==0]
  Bajando -> Subiendo_hasta_arriba [order 4] : [UI==2]
  (default) -> Idle
  Idle -> Subiendo_hasta_arriba [order 2] : [UI==2&&S<5]
  Idle -> Subiendo [order 1] : [UI == 1&&S<5]
  Subiendo -> Idle [order 1] : [S>=5||UI==0]
  Subiendo_hasta_arriba -> Idle [order 1] : [S >=5]
  Subiendo_hasta_arriba -> Subiendo [order 2] : [UI ==1]
  Subiendo -> Subiendo_hasta_arriba [order 2] : [UI==2]
  data: S input; UI input; W output double; PosMinW3 input

== stateflow chart c00021M_harness/M011/Cyber/WL/Chart ==
  state Bajand_hasta_abajo
    entry: W = -1;
  state Bajando
    entry: W = -1;
  state Idle
    entry:W = 0;
  state Subiendo_hasta_arriba
    entry: W = 1;
  state Subiendo
    entry: W = 1;
  Subiendo -> Bajand_hasta_abajo [order 4] : [UI==4]
  Bajand_hasta_abajo -> Bajando [order 2] : [UI==3]
  Subiendo -> Bajando [order 3] : [UI==3]
  Bajando -> Bajand_hasta_abajo [order 2] : [UI==4]
  Idle -> Bajando [order 3] : [UI==3&&S>0]
  Subiendo_hasta_arriba -> Bajand_hasta_abajo [order 3] : [UI==4]
  Idle -> Bajand_hasta_abajo [order 4] : [UI==4&&S>0]
  Bajando -> Subiendo [order 3] : [UI==1]
  Subiendo_hasta_arriba -> Bajando [order 4] : [UI==3]
  Bajand_hasta_abajo -> Subiendo [order 4] : [UI==1]
  Bajand_hasta_abajo -> Idle [order 1] : [S<=0]
  Bajand_hasta_abajo -> Subiendo_hasta_arriba [order 3] : [UI==2]
  Bajando -> Idle [order 1] : [S<=0||UI==0]
  Bajando -> Subiendo_hasta_arriba [order 4] : [UI==2]
  (default) -> Idle
  Idle -> Subiendo_hasta_arriba [order 2] : [UI==2&&S<5]
  Idle -> Subiendo [order 1] : [UI == 1&&S<5]
  Subiendo -> Idle [order 1] : [S>=5||UI==0]
  Subiendo_hasta_arriba -> Idle [order 1] : [S >=5]
  Subiendo_hasta_arriba -> Subiendo [order 2] : [UI ==1]
  Subiendo -> Subiendo_hasta_arriba [order 2] : [UI==2]
  data: S input; UI input; W output double

== stateflow chart c00021M_harness/M011/Cyber/WL1/Chart1 ==
  state Bajand_hasta_abajo
    entry: W = -1;
  state Bajando
    entry: W = -1;
  state Idle
    entry:W = 0;
  state Subiendo_hasta_arriba
    entry: W = 1;
  state Subiendo
    entry: W = 1;
  Subiendo -> Bajand_hasta_abajo [order 4] : [UI==4]
  Bajand_hasta_abajo -> Bajando [order 2] : [UI==3]
  Subiendo -> Bajando [order 3] : [UI==3]
  Bajando -> Bajand_hasta_abajo [order 2] : [UI==4]
  Idle -> Bajando [order 3] : [UI==3&&S>0]
  Subiendo_hasta_arriba -> Bajand_hasta_abajo [order 3] : [UI==4]
  Idle -> Bajand_hasta_abajo [order 4] : [UI==4&&S>0]
  Bajando -> Subiendo [order 3] : [UI==1]
  Subiendo_hasta_arriba -> Bajando [order 4] : [UI==3]
  Bajand_hasta_abajo -> Subiendo [order 4] : [UI==1]
  Bajand_hasta_abajo -> Idle [order 1] : [S<=0]
  Bajand_hasta_abajo -> Subiendo_hasta_arriba [order 3] : [UI==2]
  Bajando -> Idle [order 1] : [S<=0||UI==0]
  Bajando -> Subiendo_hasta_arriba [order 4] : [UI==2]
  (default) -> Idle
  Idle -> Subiendo_hasta_arriba [order 2] : [UI==2&&S<5]
  Idle -> Subiendo [order 1] : [UI == 1&&S<5]
  Subiendo -> Idle [order 1] : [S>=5||UI==0]
  Subiendo_hasta_arriba -> Idle [order 1] : [S >=5]
  Subiendo_hasta_arriba -> Subiendo [order 2] : [UI ==1]
  Subiendo -> Subiendo_hasta_arriba [order 2] : [UI==2]
  data: S input; UI input; W output double

== stateflow chart c00021M_harness/M011/Cyber/WL2/Chart1 ==
  state Bajand_hasta_abajo
    entry: W = -1;
  state Bajando
    entry: W = -1;
  state Idle
    entry:W = 0;
  state Subiendo_hasta_arriba
    entry: W = 1;
  state Subiendo
    entry: W = 1;
  Subiendo -> Bajand_hasta_abajo [order 4] : [UI==4]
  Bajand_hasta_abajo -> Bajando [order 2] : [UI==3]
  Subiendo -> Bajando [order 3] : [UI==3]
  Bajando -> Bajand_hasta_abajo [order 2] : [UI==4]
  Idle -> Bajando [order 3] : [UI==3&&S>PosMinW3]
  Subiendo_hasta_arriba -> Bajand_hasta_abajo [order 3] : [UI==4]
  Idle -> Bajand_hasta_abajo [order 4] : [UI==4&&S>PosMinW3]
  Bajando -> Subiendo [order 3] : [UI==1]
  Subiendo_hasta_arriba -> Bajando [order 4] : [UI==3]
  Bajand_hasta_abajo -> Subiendo [order 4] : [UI==1]
  Bajand_hasta_abajo -> Idle [order 1] : [S<=PosMinW3]
  Bajand_hasta_abajo -> Subiendo_hasta_arriba [order 3] : [UI==2]
  Bajando -> Idle [order 1] : [S<=PosMinW3||UI==0]
  Bajando -> Subiendo_hasta_arriba [order 4] : [UI==2]
  (default) -> Idle
  Idle -> Subiendo_hasta_arriba [order 2] : [UI==2&&S<5]
  Idle -> Subiendo [order 1] : [UI == 1&&S<5]
  Subiendo -> Idle [order 1] : [S>=5||UI==0]
  Subiendo_hasta_arriba -> Idle [order 1] : [S >=5]
  Subiendo_hasta_arriba -> Subiendo [order 2] : [UI ==1]
  Subiendo -> Subiendo_hasta_arriba [order 2] : [UI==2]
  data: S input; UI input; W output double; PosMinW3 input

== stateflow chart c00021M_harness/M012/Cyber/WL/Chart ==
  state Bajand_hasta_abajo
    entry: W = -1;
  state Bajando
    entry: W = -1;
  state Idle
    entry:W = 0;
  state Subiendo_hasta_arriba
    entry: W = 1;
  state Subiendo
    entry: W = 1;
  Subiendo -> Bajand_hasta_abajo [order 4] : [UI==4]
  Bajand_hasta_abajo -> Bajando [order 2] : [UI==3]
  Subiendo -> Bajando [order 3] : [UI==3]
  Bajando -> Bajand_hasta_abajo [order 2] : [UI==4]
  Idle -> Bajando [order 3] : [UI==3&&S>0]
  Subiendo_hasta_arriba -> Bajand_hasta_abajo [order 3] : [UI==4]
  Idle -> Bajand_hasta_abajo [order 4] : [UI==4&&S>0]
  Bajando -> Subiendo [order 3] : [UI==1]
  Subiendo_hasta_arriba -> Bajando [order 4] : [UI==3]
  Bajand_hasta_abajo -> Subiendo [order 4] : [UI==1]
  Bajand_hasta_abajo -> Idle [order 1] : [S<=0]
  Bajand_hasta_abajo -> Subiendo_hasta_arriba [order 3] : [UI==2]
  Bajando -> Idle [order 1] : [S<=0||UI==0]
  Bajando -> Subiendo_hasta_arriba [order 4] : [UI==2]
  (default) -> Idle
  Idle -> Subiendo_hasta_arriba [order 2] : [UI==2&&S<5]
  Idle -> Subiendo [order 1] : [UI == 1&&S<5]
  Subiendo -> Idle [order 1] : [S>=5||UI==0]
  Subiendo_hasta_arriba -> Idle [order 1] : [S >=5]
  Subiendo_hasta_arriba -> Subiendo [order 2] : [UI ==1]
  Subiendo -> Subiendo_hasta_arriba [order 2] : [UI==2]
  data: S input; UI input; W output double

== stateflow chart c00021M_harness/M012/Cyber/WL1/Chart1 ==
  state Bajand_hasta_abajo
    entry: W = -1;
  state Bajando
    entry: W = -1;
  state Idle
    entry:W = 0;
  state Subiendo_hasta_arriba
    entry: W = 1;
  state Subiendo
    entry: W = 1;
  Subiendo -> Bajand_hasta_abajo [order 4] : [UI==4]
  Bajand_hasta_abajo -> Bajando [order 2] : [UI==3]
  Subiendo -> Bajando [order 3] : [UI==3]
  Bajando -> Bajand_hasta_abajo [order 2] : [UI==4]
  Idle -> Bajando [order 3] : [UI==3&&S>0]
  Subiendo_hasta_arriba -> Bajand_hasta_abajo [order 3] : [UI==4]
  Idle -> Bajand_hasta_abajo [order 4] : [UI==4&&S>0]
  Bajando -> Subiendo [order 3] : [UI==1]
  Subiendo_hasta_arriba -> Bajando [order 4] : [UI==3]
  Bajand_hasta_abajo -> Subiendo [order 4] : [UI==1]
  Bajand_hasta_abajo -> Idle [order 1] : [S<=0]
  Bajand_hasta_abajo -> Subiendo_hasta_arriba [order 3] : [UI==2]
  Bajando -> Idle [order 1] : [S<=0||UI==0]
  Bajando -> Subiendo_hasta_arriba [order 4] : [UI==2]
  (default) -> Idle
  Idle -> Subiendo_hasta_arriba [order 2] : [UI==2&&S<5]
  Idle -> Subiendo [order 1] : [UI == 1&&S<5]
  Subiendo -> Idle [order 1] : [S>=5||UI==0]
  Subiendo_hasta_arriba -> Idle [order 1] : [S >=5]
  Subiendo_hasta_arriba -> Subiendo [order 2] : [UI ==1]
  Subiendo -> Subiendo_hasta_arriba [order 2] : [UI==2]
  data: S input; UI input; W output double

== stateflow chart c00021M_harness/M012/Cyber/WL2/Chart1 ==
  state Bajand_hasta_abajo
    entry: W = -1;
  state Bajando
    entry: W = -1;
  state Idle
    entry:W = 0;
  state Subiendo_hasta_arriba
    entry: W = 1;
  state Subiendo
    entry: W = 1;
  Subiendo -> Bajand_hasta_abajo [order 4] : [UI==4]
  Bajand_hasta_abajo -> Bajando [order 2] : [UI==3]
  Subiendo -> Bajando [order 3] : [UI==3]
  Bajando -> Bajand_hasta_abajo [order 2] : [UI==4]
  Idle -> Bajando [order 3] : [UI==3&&S>PosMinW3]
  Subiendo_hasta_arriba -> Bajand_hasta_abajo [order 3] : [UI==4]
  Idle -> Bajand_hasta_abajo [order 4] : [UI==4&&S>PosMinW3]
  Bajando -> Subiendo [order 3] : [UI==1]
  Subiendo_hasta_arriba -> Bajando [order 4] : [UI==3]
  Bajand_hasta_abajo -> Subiendo [order 4] : [UI==1]
  Bajand_hasta_abajo -> Idle [order 1] : [S<=PosMinW3]
  Bajand_hasta_abajo -> Subiendo_hasta_arriba [order 3] : [UI==2]
  Bajando -> Idle [order 1] : [S<=PosMinW3||UI==0]
  Bajando -> Subiendo_hasta_arriba [order 4] : [UI==2]
  (default) -> Idle
  Idle -> Subiendo_hasta_arriba [order 2] : [UI==2&&S<5]
  Idle -> Subiendo [order 1] : [UI == 1&&S<5]
  Subiendo -> Idle [order 1] : [S>=5||UI==0]
  Subiendo_hasta_arriba -> Idle [order 1] : [S >=5]
  Subiendo_hasta_arriba -> Subiendo [order 2] : [UI ==1]
  Subiendo -> Subiendo_hasta_arriba [order 2] : [UI==2]
  data: S input; UI input; W output double; PosMinW3 input

== stateflow chart c00021M_harness/M013/Cyber/WL/Chart ==
  state Bajand_hasta_abajo
    entry: W = -1;
  state Bajando
    entry: W = -1;
  state Idle
    entry:W = 0;
  state Subiendo_hasta_arriba
    entry: W = 1;
  state Subiendo
    entry: W = 1;
  Subiendo -> Bajand_hasta_abajo [order 4] : [UI==4]
  Bajand_hasta_abajo -> Bajando [order 2] : [UI==3]
  Subiendo -> Bajando [order 3] : [UI==3]
  Bajando -> Bajand_hasta_abajo [order 2] : [UI==4]
  Idle -> Bajando [order 3] : [UI==3&&S>0]
  Subiendo_hasta_arriba -> Bajand_hasta_abajo [order 3] : [UI==4]
  Idle -> Bajand_hasta_abajo [order 4] : [UI==4&&S>0]
  Bajando -> Subiendo [order 3] : [UI==1]
  Subiendo_hasta_arriba -> Bajando [order 4] : [UI==3]
  Bajand_hasta_abajo -> Subiendo [order 4] : [UI==1]
  Bajand_hasta_abajo -> Idle [order 1] : [S<=0]
  Bajand_hasta_abajo -> Subiendo_hasta_arriba [order 3] : [UI==2]
  Bajando -> Idle [order 1] : [S<=0||UI==0]
  Bajando -> Subiendo_hasta_arriba [order 4] : [UI==2]
  (default) -> Idle
  Idle -> Subiendo_hasta_arriba [order 2] : [UI==2&&S<5]
  Idle -> Subiendo [order 1] : [UI == 1&&S<5]
  Subiendo -> Idle [order 1] : [S>=5||UI==0]
  Subiendo_hasta_arriba -> Idle [order 1] : [S >=5]
  Subiendo_hasta_arriba -> Subiendo [order 2] : [UI ==1]
  Subiendo -> Subiendo_hasta_arriba [order 2] : [UI==2]
  data: S input; UI input; W output double

== stateflow chart c00021M_harness/M013/Cyber/WL1/Chart1 ==
  state Bajand_hasta_abajo
    entry: W = -1;
  state Bajando
    entry: W = -1;
  state Idle
    entry:W = 0;
  state Subiendo_hasta_arriba
    entry: W = 1;
  state Subiendo
    entry: W = 1;
  Subiendo -> Bajand_hasta_abajo [order 4] : [UI==4]
  Bajand_hasta_abajo -> Bajando [order 2] : [UI==3]
  Subiendo -> Bajando [order 3] : [UI==3]
  Bajando -> Bajand_hasta_abajo [order 2] : [UI==4]
  Idle -> Bajando [order 3] : [UI==3&&S>0]
  Subiendo_hasta_arriba -> Bajand_hasta_abajo [order 3] : [UI==4]
  Idle -> Bajand_hasta_abajo [order 4] : [UI==4&&S>0]
  Bajando -> Subiendo [order 3] : [UI==1]
  Subiendo_hasta_arriba -> Bajando [order 4] : [UI==3]
  Bajand_hasta_abajo -> Subiendo [order 4] : [UI==1]
  Bajand_hasta_abajo -> Idle [order 1] : [S<=0]
  Bajand_hasta_abajo -> Subiendo_hasta_arriba [order 3] : [UI==2]
  Bajando -> Idle [order 1] : [S<=0||UI==0]
  Bajando -> Subiendo_hasta_arriba [order 4] : [UI==2]
  (default) -> Idle
  Idle -> Subiendo_hasta_arriba [order 2] : [UI==2&&S<5]
  Idle -> Subiendo [order 1] : [UI == 1&&S<5]
  Subiendo -> Idle [order 1] : [S>=5||UI==0]
  Subiendo_hasta_arriba -> Idle [order 1] : [S >=5]
  Subiendo_hasta_arriba -> Subiendo [order 2] : [UI ==1]
  Subiendo -> Subiendo_hasta_arriba [order 2] : [UI==2]
  data: S input; UI input; W output double

== stateflow chart c00021M_harness/M013/Cyber/WL2/Chart1 ==
  state Bajand_hasta_abajo
    entry: W = -1;
  state Bajando
    entry: W = -1;
  state Idle
    entry:W = 0;
  state Subiendo_hasta_arriba
    entry: W = 1;
  state Subiendo
    entry: W = 1;
  Subiendo -> Bajand_hasta_abajo [order 4] : [UI==4]
  Bajand_hasta_abajo -> Bajando [order 2] : [UI==3]
  Subiendo -> Bajando [order 3] : [UI==3]
  Bajando -> Bajand_hasta_abajo [order 2] : [UI==4]
  Idle -> Bajando [order 3] : [UI==3&&S>PosMinW3]
  Subiendo_hasta_arriba -> Bajand_hasta_abajo [order 3] : [UI==4]
  Idle -> Bajand_hasta_abajo [order 4] : [UI==4&&S>PosMinW3]
  Bajando -> Subiendo [order 3] : [UI==1]
  Subiendo_hasta_arriba -> Bajando [order 4] : [UI==3]
  Bajand_hasta_abajo -> Subiendo [order 4] : [UI==1]
  Bajand_hasta_abajo -> Idle [order 1] : [S<=PosMinW3]
  Bajand_hasta_abajo -> Subiendo_hasta_arriba [order 3] : [UI==2]
  Bajando -> Idle [order 1] : [S<=PosMinW3||UI==0]
  Bajando -> Subiendo_hasta_arriba [order 4] : [UI==2]
  (default) -> Idle
  Idle -> Subiendo_hasta_arriba [order 2] : [UI==2&&S<5]
  Idle -> Subiendo [order 1] : [UI == 1&&S<5]
  Subiendo -> Idle [order 1] : [S>=5||UI==0]
  Subiendo_hasta_arriba -> Idle [order 1] : [S >=5]
  Subiendo_hasta_arriba -> Subiendo [order 2] : [UI ==1]
  Subiendo -> Subiendo_hasta_arriba [order 2] : [UI==2]
  data: S input; UI input; W output double; PosMinW3 input

== stateflow chart c00021M_harness/M015/Cyber/WL/Chart ==
  state Bajand_hasta_abajo
    entry: W = -1;
  state Bajando
    entry: W = 0;
  state Idle
    entry:W = 0;
  state Subiendo_hasta_arriba
    entry: W = 1;
  state Subiendo
    entry: W = 1;
  Subiendo -> Bajand_hasta_abajo [order 4] : [UI==4]
  Bajand_hasta_abajo -> Bajando [order 2] : [UI==3]
  Subiendo -> Bajando [order 3] : [UI==3]
  Bajando -> Bajand_hasta_abajo [order 2] : [UI==4]
  Idle -> Bajando [order 3] : [UI==3&&S>0]
  Subiendo_hasta_arriba -> Bajand_hasta_abajo [order 3] : [UI==4]
  Idle -> Bajand_hasta_abajo [order 4] : [UI==4&&S>0]
  Bajando -> Subiendo [order 3] : [UI==1]
  Subiendo_hasta_arriba -> Bajando [order 4] : [UI==3]
  Bajand_hasta_abajo -> Subiendo [order 4] : [UI==1]
  Bajand_hasta_abajo -> Idle [order 1] : [S<=0]
  Bajand_hasta_abajo -> Subiendo_hasta_arriba [order 3] : [UI==2]
  Bajando -> Idle [order 1] : [S<=0||UI==0]
  Bajando -> Subiendo_hasta_arriba [order 4] : [UI==2]
  (default) -> Idle
  Idle -> Subiendo_hasta_arriba [order 2] : [UI==2&&S<5]
  Idle -> Subiendo [order 1] : [UI == 1&&S<5]
  Subiendo -> Idle [order 1] : [S>=5||UI==0]
  Subiendo_hasta_arriba -> Idle [order 1] : [S >=5]
  Subiendo_hasta_arriba -> Subiendo [order 2] : [UI ==1]
  Subiendo -> Subiendo_hasta_arriba [order 2] : [UI==2]
  data: S input; UI input; W output double
